simulink model "Filtro_teste_corrente_constante"  (R2014a)
settings: Solver=ode45  StartTime=0.0  StopTime=0.08  MaxStep=1e-6  RelTol=1e-3
libraries: powerlib x36, dsparch4 x4, powerlib_meascontrol x4, simulink x2, sps_avr x1
settings Model: Creator=JPSOLIV  LastModifiedBy=Joao
settings SolverCC: AlgebraicLoopSolver=LineSearch
settings DebuggingCC: MergeDetectMultiDrivingBlocksExec=error

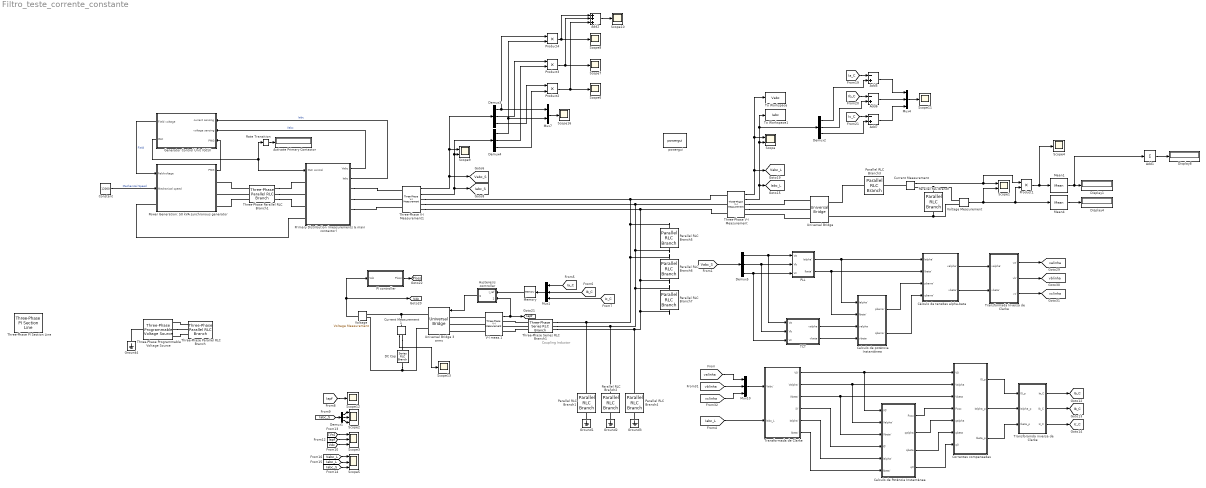
== system Filtro_teste_corrente_constante ==
  note: Coupling Inductor
  Activate Primary Contactor : Display
      settings: SampleTime=1e-2
  Add1 : Sum  Inputs=+
  Add2 : Sum  Inputs=+++
  Add5 : Sum  Inputs=-+
  Add6 : Sum  Inputs=-+
  Add7 : Sum  Inputs=-+
  Calculo de Potência Instantânea : Subsystem
  Calculo de potência Instantânea : Subsystem
  Constant : Constant  Value=12000
  Correntes compensadas : Subsystem
  Current Measurement : powerlib/Measurements/Current Measurement  PhasorSimulation=off  OutputType=Complex  PSBequivalent=0
  Current Measurement1 : powerlib/Measurements/Current Measurement  PhasorSimulation=off  OutputType=Complex  PSBequivalent=0
  Cálculo de tensões alpha-beta : Subsystem
  DC Cap : powerlib/Elements/Series RLC Branch  LConnTagsString=__new0  RConnTagsString=__new0  BranchType=C  Resistance=1  Inductance=1e-3  SetiL0=off  InitialCurrent=0  Capacitance=100e-6  Setx0=off  InitialVoltage=4000  Measurements=None
  Demux{1..5} (5 alike) : Demux  Outputs=3
  Display1 : Display
  Display4 : Display
  Display8 : Display
  Generator Control Unit (GCU) : Subsystem
      mask Display: image(imread('power_aircraft_distribution_GCU.jpg','jpg'))
  Ground{1..4} (4 alike) : powerlib/Elements/Ground  LConnTagsString=a
  Hysteresis controller : Subsystem
  Mean1 : powerlib_meascontrol/Measurements/Mean  Freq=400  Vinit=0  Ts=0
  Mean4 : powerlib_meascontrol/Measurements/Mean  Freq=400  Vinit=0  Ts=0
  Memory : Memory
  Mux1 : Mux  Inputs=3
  Mux10 : Mux  Inputs=3
  Mux4 : Mux  Inputs=3
  Mux7 : Mux  Inputs=2
  PI controller : Subsystem
  PLL : Subsystem
  Parallel RLC Branch : powerlib/Elements/Parallel RLC Branch  LConnTagsString=a  RConnTagsString=__new0  BranchType=RC  Resistance=50  Inductance=1e-3  SetiL0=off  InitialCurrent=0  Capacitance=30e-6  Setx0=off  InitialVoltage=0  Measurements=None
  Parallel RLC Branch1 : powerlib/Elements/Parallel RLC Branch  LConnTagsString=a  RConnTagsString=__new0  BranchType=RC  Resistance=10e3  Inductance=1e-3  SetiL0=off  InitialCurrent=0  Capacitance=3.9789e-08  Setx0=off  InitialVoltage=0  Measurements=None
  Parallel RLC Branch2 : powerlib/Elements/Parallel RLC Branch  LConnTagsString=a  RConnTagsString=__new0  BranchType=RC  Resistance=10e3  Inductance=1e-3  SetiL0=off  InitialCurrent=0  Capacitance=3.9789e-08  Setx0=off  InitialVoltage=0  Measurements=None
  Parallel RLC Branch3 : powerlib/Elements/Parallel RLC Branch  LConnTagsString=a  RConnTagsString=__new0  BranchType=L  Resistance=1  Inductance=10e-3  SetiL0=off  InitialCurrent=0  Capacitance=30e-6  Setx0=off  InitialVoltage=0  Measurements=None
  Parallel RLC Branch4 : powerlib/Elements/Parallel RLC Branch  LConnTagsString=a  RConnTagsString=__new0  BranchType=RC  Resistance=10e3  Inductance=1e-3  SetiL0=off  InitialCurrent=0  Capacitance=3.9789e-08  Setx0=off  InitialVoltage=0  Measurements=None
  Parallel RLC Branch5 : powerlib/Elements/Parallel RLC Branch  LConnTagsString=a  RConnTagsString=__new0  BranchType=C  Resistance=10e3  Inductance=1e-3  SetiL0=off  InitialCurrent=0  Capacitance=.1e-6  Setx0=off  InitialVoltage=0  Measurements=None
  Parallel RLC Branch6 : powerlib/Elements/Parallel RLC Branch  LConnTagsString=a  RConnTagsString=__new0  BranchType=C  Resistance=10e3  Inductance=1e-3  SetiL0=off  InitialCurrent=0  Capacitance=.1e-6  Setx0=off  InitialVoltage=0  Measurements=None
  Parallel RLC Branch7 : powerlib/Elements/Parallel RLC Branch  LConnTagsString=a  RConnTagsString=__new0  BranchType=C  Resistance=10e3  Inductance=1e-3  SetiL0=off  InitialCurrent=0  Capacitance=.1e-6  Setx0=off  InitialVoltage=0  Measurements=None
  Power Generation: 50 kVA synchronous generator : Subsystem
      mask Display: image(imread('power_aircraft_distribution_APU_Generator.jpg','jpg'))
  Primary Distribution (measurements & main contactor) : Subsystem
  Product{1..4} (4 alike) : Product
  Rate Transition : RateTransition  OutPortSampleTimeOpt=Inherit  OutPortSampleTime=Ts
  Scope : Scope  NumInputPorts=2
      settings: YMin=-200~-25  YMax=200~25
  Scope1 : Scope  NumInputPorts=2
      settings: YMin=-0.00561601~0  YMax=20~500
  Scope{4,6..8,10..13,16} (9 alike) : Scope
      Scope10 settings: YMin=-2000  YMax=16000  SaveName=ScopeData18
      Scope11 settings: YMin=-60  YMax=60  SaveName=ScopeData11
      Scope12 settings: YMin=-150  YMax=200  SaveName=ScopeData12
      Scope13 settings: YMin=-20  YMax=70  SaveName=ScopeData31
      Scope16 settings: YMin=-250  YMax=450  SaveName=ScopeData17
      Scope4 settings: YMin=0  YMax=8000  SaveName=ScopeData2
      Scope6 settings: YMin=-1000  YMax=6000  SaveName=ScopeData7
      Scope7 settings: YMin=-1000  YMax=6000  SaveName=ScopeData13
      Scope8 settings: YMin=-10000  YMax=15000  SaveName=ScopeData14
  Scope2 : Scope  NumInputPorts=3
      settings: TimeRange=0.015  YMin=-40~-40~-40  YMax=40~40~40  SaveName=Isource  MaxDataPoints=500000
  Scope3 : Scope  NumInputPorts=3
      settings: TimeRange=0.015  YMin=-1~-20~275  YMax=1~20~575  SaveName=Vs_Iapf_Vdc  MaxDataPoints=500000
  Scope5 : Scope  NumInputPorts=3
      settings: TimeRange=0.015  YMin=-200~-6~-10  YMax=200~6~10  SaveName=Vs_Iapf_Vdc1  MaxDataPoints=500000
  Scope9 : Scope  NumInputPorts=2
      settings: YMin=-175~-7  YMax=175~7  SaveName=ScopeData9
  TCT : Subsystem
  Three-Phase PI Section Line : powerlib/Elements/Three-Phase PI Section Line  LConnTagsString=a|b|c  RConnTagsString=A|B|C  Frequency=400  Resistances=[ 0.01273 0.3864]  Inductances="[ 0.9337e-3  4.1264e-3]"  Capacitances=[12.74e-9 7.751e-9]  Length=0.005
  Three-Phase Parallel RLC Branch : powerlib/Elements/Three-Phase Parallel RLC Branch  LConnTagsString=A|B|C  RConnTagsString=A|B|C  BranchType=RL  Resistance=0.0367e-3  Inductance=6e-6  Capacitance=1e-6  Measurements=None
  Three-Phase Parallel RLC Branch1 : powerlib/Elements/Three-Phase Parallel RLC Branch  LConnTagsString=A|B|C  RConnTagsString=A|B|C  BranchType=RL  Resistance=0.367  Inductance=6e-3  Capacitance=1e-6  Measurements=None
  Three-Phase Programmable Voltage Source : powerlib/Electrical Sources/Three-Phase Programmable Voltage Source  PositiveSequence="[115*sqrt(3)  0 400]"  VariationEntity=None  VariationType=Table of time-amplitude pairs  VariationTypeAlt=Step  VariationStep=0.5  VariationRate=10  VariationMagnitude=0.3  VariationFrequency=2  VariationTiming=[1 2]  VariationPhaseA=off  Amplitudes=[1 0.8 1.2 1.0]  TimeValues=[0 0.1 0.15 0.2]  HarmonicGeneration=off  HarmonicA=[3 0.2 -25 0]  HarmonicB=[2 0.15 35 2]  Timing="[0.05  3]"  BusType=swing  Pref=0  Qref=0  Qmin=-inf  Qmax=inf
  Three-Phase Series RLC Branch1 : powerlib/Elements/Three-Phase Series RLC Branch  LConnTagsString=A|B|C  RConnTagsString=A|B|C  BranchType=L  Resistance=1e9  Inductance=5e-4  Capacitance=.2e-3  Measurements=None
  Three-Phase V-I Measurement : powerlib/Measurements/Three-Phase V-I Measurement  VoltageMeasurement=phase-to-ground  SetLabelV=off  LabelV=Vabc  Vpu=off  VpuLL=off  CurrentMeasurement=yes  SetLabelI=off  LabelI=Iabc  Ipu=off  Pbase=100e6  Vbase=500e3  OutputType=Complex  PhasorSimulation=off  PSBequivalent=0
  Three-Phase V-I Measurement1 : powerlib/Measurements/Three-Phase V-I Measurement  VoltageMeasurement=phase-to-ground  SetLabelV=off  LabelV=Vabc  Vpu=off  VpuLL=off  CurrentMeasurement=yes  SetLabelI=off  LabelI=Iabc  Ipu=off  Pbase=100e6  Vbase=500e3  OutputType=Complex  PhasorSimulation=off  PSBequivalent=0
  To Workspace : ToWorkspace  VariableName=Vabc  SaveFormat=Structure With Time  SampleTime=-1
  To Workspace1 : ToWorkspace  VariableName=Iabc  SaveFormat=Structure With Time  SampleTime=-1
  Transforamda inversa de Clarke : Subsystem
  Transformada Inversa de Clarke : Subsystem
  Transformada de Clarke : Subsystem
  Universal Bridge : powerlib/Power Electronics/Universal Bridge  Arms=3  SnubberResistance=1e5  SnubberCapacitance=inf  Device=Diodes  Ron=1e-3  Lon=0  ForwardVoltages="[  0  0  ]"  ForwardVoltage=0  GTOparameters=[ 10e-6 , 20e-6 ]  IGBTparameters=[ 1e-6 , 2e-6 ]  Measurements=None  Measurements_2=None  converterType=Rectifier
  Universal Bridge 3 arms : powerlib/Power Electronics/Universal Bridge  Arms=3  SnubberResistance=10000  SnubberCapacitance=inf  Device=IGBT / Diodes  Ron=1e-4  Lon=0  ForwardVoltages="[  1  1  ]"  ForwardVoltage=.8  GTOparameters=[ 10e-6 , 20e-6 ]  IGBTparameters=[ 1e-6 , 2e-6 ]  Measurements=None  Measurements_2=None  converterType=Rectifier
  V-I meas.1 : powerlib/Measurements/Three-Phase V-I Measurement  VoltageMeasurement=phase-to-phase  SetLabelV=on  LabelV=Vnm  Vpu=off  VpuLL=off  CurrentMeasurement=yes  SetLabelI=off  LabelI=Iabc  Ipu=off  Pbase=100e6  Vbase=500e3  OutputType=Complex  PhasorSimulation=off  PSBequivalent=0
  Voltage : powerlib/Measurements/Voltage Measurement  PhasorSimulation=off  OutputType=Complex  PSBequivalent=0
  Voltage Measurement : powerlib/Measurements/Voltage Measurement  PhasorSimulation=off  OutputType=Complex  PSBequivalent=0
  powergui : powerlib/powergui  Priority=1  SimulationMode=Discrete  SolverType=Tustin  SampleTime=1e-7  frequency=60  SPID=off  DisableSnubberDevices=off  DisableRonSwitches=off  DisableVfSwitches=off  SwTol=0  Interpol=off  DisplayEquations=off  Ts=100  methode=off  frequencyindice=400  Pbase=100e6  ErrMax=1e-4  Iterations=50  UnitsV=kV  UnitsW=MW  FunctionMessages=off  echomessages=off  HookPort=off  EnableUseOfTLC=off  x0status=blocks  RestoreLinks=warning  ResistiveCurrentMeasurement=off  Frange=[0:2:500]  Ylog=off  Xlog=on  ShowGrid=off  save=off  variable=ZData  structure=0  ZoomFFT=off  StartTime=0.0  cycles=1  DisplayStyle=1  fundamental=60  FreqAxis=off  MaxFrequency=1000  frequencyindicesteady=1  RmsSteady=1  display=off
  tag scope: Ia_C=global, Iabc_L=global, Iabc_S=global, Iapf=global, Ib_C=global, Ic_C=global, Ploss=global, Vabc_L=global, Vabc_S=global, Vdc=global, valinha=global, vblinha=global, vclinha=global
  wires:
  Three-Phase V-I Measurement/1 -> [Vabc_L], To Workspace/1, Scope/1
  Three-Phase V-I Measurement/2 -> [Iabc_L], Demux2/1, To Workspace1/1, Scope/2
  [Ia_C] -> Add5/1
  [Ib_C] -> Add6/1
  [Ic_C] -> Add7/1
  Demux2/1 -> Add5/2
  Demux2/2 -> Add6/2
  Demux2/3 -> Add7/2
  Add6/1 -> Mux4/2
  Mux4/1 -> Scope11/1
  Add7/1 -> Mux4/3
  Add5/1 -> Mux4/1
  Current Measurement/1 -> Product1/1, Scope1/1
  Voltage Measurement/1 -> Scope1/2, Product1/2, Mean4/1
  Product1/1 -> Scope4/1, Mean1/1
  Mean1/1 -> Add1/1, Display1/1
  Mean4/1 -> Display4/1
  Add1/1 -> Display8/1
  Three-Phase V-I Measurement1/1 -> [Vabc_S], Demux3/1, Scope9/1
  Three-Phase V-I Measurement1/2 -> [Iabc_S], Demux4/1, Scope9/2
  Demux3/1 -> Mux7/1, Product4/1
  Mux7/1 -> Scope16/1
  Transformada de Clarke/1(V0') -> Calculo de Potência Instantânea/1(V0'), Correntes compensadas/1(V0)
  Correntes compensadas/2(Ialpha_p) -> Transforamda inversa de Clarke/2(Ialpha_p)
  Correntes compensadas/3(Ibeta_p) -> Transforamda inversa de Clarke/3(Ibeta_p)
  Voltage/1 -> [Vdc], PI controller/1(Vdc)
  PI controller/1(Ploss) -> [Ploss]
  Transforamda inversa de Clarke/1(Ia_C) -> [Ia_C]
  Transforamda inversa de Clarke/2(Ib_C) -> [Ib_C]
  Transforamda inversa de Clarke/3(Ic_C) -> [Ic_C]
  [Iapf] -> Scope12/1
  Demux1/1 -> Scope2/1
  Demux1/2 -> Scope2/2
  Demux1/3 -> Scope2/3
  [Iabc_S] -> Demux1/1
  [Vs] -> Scope3/1
  [Vdc] -> Scope3/3
  [Iapf] -> Scope3/2
  [Vabc_L] -> Scope5/1
  [Iabc_S] -> Scope5/3
  [Iabc_L] -> Scope5/2
  Product2/1 -> Add2/3, Scope6/1
  Power Generation: 50 kVA synchronous generator/1(PMG) -> Generator Control Unit (GCU)/3(PMG)
  Generator Control Unit (GCU)/1(Field voltage) -> Power Generation: 50 kVA synchronous generator/1(fieldvoltage)  "Field"
  Primary Distribution (measurements & main contactor)/1(Vabc) -> Generator Control Unit (GCU)/2(voltage sensing)  "Vabc"
  Primary Distribution (measurements & main contactor)/2(Iabc) -> Generator Control Unit (GCU)/1(current sensing)  "Iabc"
  Generator Control Unit (GCU)/2(GLC) -> Primary Distribution (measurements & main contactor)/1(GLC control), Rate Transition/1
  Constant/1 -> Power Generation: 50 kVA synchronous generator/2(Mechanical speed)  "Mechanical Speed"
  Rate Transition/1 -> Activate Primary Contactor/1
  V-I meas.1/1 -> Hysteresis controller/2(I_meas), [Iapf]
  Mux1/1 -> Memory/1
  Hysteresis controller/1(g) -> Universal Bridge 3 arms/1
  [Ia_C] -> Mux1/1
  [Ib_C] -> Mux1/2
  [Ic_C] -> Mux1/3
  Memory/1 -> Hysteresis controller/1(I_ref)
  Product3/1 -> Add2/2, Scope7/1
  Demux4/1 -> Mux7/2, Product4/2
  Demux3/2 -> Product3/1
  Demux4/2 -> Product3/2
  Demux3/3 -> Product2/1
  Demux4/3 -> Product2/2
  Product4/1 -> Scope8/1, Add2/1
  Add2/1 -> Scope10/1
  [Vabc_S] -> Demux5/1
  [valinha] -> Mux10/1
  [vblinha] -> Mux10/2
  [vclinha] -> Mux10/3
  Mux10/1 -> Transformada de Clarke/1(Vabc')
  [Iabc_L] -> Transformada de Clarke/2(Iabc_L)
  Transformada de Clarke/2(Valpha') -> Calculo de Potência Instantânea/2(Valpha'), Correntes compensadas/2(Valpha)
  Transformada de Clarke/3(Vbeta') -> Calculo de Potência Instantânea/3(Vbeta'), Correntes compensadas/3(Vbeta)
  Transformada de Clarke/4(i0') -> Calculo de Potência Instantânea/4(I0')
  Transformada de Clarke/5(Ialpha') -> Calculo de Potência Instantânea/5(Ialpha')
  Transformada de Clarke/6(Ibeta') -> Calculo de Potência Instantânea/6(Ibeta')
  Calculo de Potência Instantânea/1(Posc) -> Correntes compensadas/4(Posc)
  Calculo de Potência Instantânea/2(qalpha) -> Correntes compensadas/5(qalpha)
  Calculo de Potência Instantânea/3(qbeta) -> Correntes compensadas/6(qbeta)
  Calculo de Potência Instantânea/4(q0) -> Correntes compensadas/7(q0)
  Correntes compensadas/1(I0_p) -> Transforamda inversa de Clarke/1(I0_p)
  Demux5/1 -> PLL/1(Va), TCT/1(Va)
  Demux5/2 -> PLL/2(Vb), TCT/2(Vb)
  Demux5/3 -> PLL/3(Vc), TCT/3(Vc)
  TCT/1(valpha) -> Calculo de potência Instantânea/3(valpha)
  TCT/2(vbeta) -> Calculo de potência Instantânea/4(vbeta)
  Calculo de potência Instantânea/2(qbarra') -> Cálculo de tensões alpha-beta/4(qbarra')
  PLL/1(Ialpha') -> Calculo de potência Instantânea/1(Ialpha'), Cálculo de tensões alpha-beta/1(Ialpha')
  PLL/2(Ibeta') -> Calculo de potência Instantânea/2(Ibeta'), Cálculo de tensões alpha-beta/2(Ibeta')
  Calculo de potência Instantânea/1(pbarra') -> Cálculo de tensões alpha-beta/3(pbarra')
  Cálculo de tensões alpha-beta/1(valpha') -> Transformada Inversa de Clarke/1(valpha')
  Cálculo de tensões alpha-beta/2(vbeta') -> Transformada Inversa de Clarke/2(vbeta')
  Transformada Inversa de Clarke/1(va') -> [valinha]
  Transformada Inversa de Clarke/2(vb') -> [vblinha]
  Transformada Inversa de Clarke/3(vc') -> [vclinha]
  Current Measurement1/1 -> Scope13/1
  connections:
  Parallel RLC Branch/RConn1 -- Universal Bridge/RConn2 -- Voltage Measurement/LConn2
  Three-Phase V-I Measurement/RConn1 -- Universal Bridge/LConn1
  Current Measurement/RConn1 -- Voltage Measurement/LConn1 -- Parallel RLC Branch/LConn1
  Parallel RLC Branch3/RConn1 -- Universal Bridge/RConn1
  Three-Phase V-I Measurement1/RConn2 -- Three-Phase V-I Measurement/LConn2 -- Parallel RLC Branch5/RConn1 -- Three-Phase Series RLC Branch1/RConn2 -- Parallel RLC Branch2/LConn1 -- Parallel RLC Branch7/LConn1
  Current Measurement/LConn1 -- Parallel RLC Branch3/LConn1
  Three-Phase V-I Measurement/RConn2 -- Universal Bridge/LConn2
  Universal Bridge/LConn3 -- Three-Phase V-I Measurement/RConn3
  Three-Phase V-I Measurement1/RConn3 -- Three-Phase V-I Measurement/LConn3 -- Parallel RLC Branch6/RConn1 -- Parallel RLC Branch4/LConn1 -- Three-Phase Series RLC Branch1/RConn3 -- Parallel RLC Branch7/RConn1
  Three-Phase V-I Measurement1/RConn1 -- Parallel RLC Branch1/LConn1 -- Three-Phase Series RLC Branch1/RConn1 -- Parallel RLC Branch6/LConn1 -- Parallel RLC Branch5/LConn1 -- Three-Phase V-I Measurement/LConn1
  Universal Bridge 3 arms/RConn1 -- Current Measurement1/LConn1 -- Voltage/LConn1
  Universal Bridge 3 arms/RConn2 -- Voltage/LConn2 -- DC Cap/RConn1
  V-I meas.1/LConn2 -- Universal Bridge 3 arms/LConn2
  V-I meas.1/LConn1 -- Universal Bridge 3 arms/LConn1
  V-I meas.1/LConn3 -- Universal Bridge 3 arms/LConn3
  Ground1/LConn1 -- Parallel RLC Branch1/RConn1
  Ground2/LConn1 -- Parallel RLC Branch2/RConn1
  Ground3/LConn1 -- Parallel RLC Branch4/RConn1
  Three-Phase Parallel RLC Branch1/RConn3 -- Primary Distribution (measurements & main contactor)/LConn3
  Three-Phase Parallel RLC Branch1/LConn1 -- Power Generation: 50 kVA synchronous generator/RConn1
  Three-Phase Parallel RLC Branch1/LConn2 -- Power Generation: 50 kVA synchronous generator/RConn2
  Power Generation: 50 kVA synchronous generator/LConn1 -- Primary Distribution (measurements & main contactor)/LConn4
  Three-Phase Parallel RLC Branch1/RConn2 -- Primary Distribution (measurements & main contactor)/LConn2
  Three-Phase Parallel RLC Branch1/LConn3 -- Power Generation: 50 kVA synchronous generator/RConn3
  Three-Phase Parallel RLC Branch1/RConn1 -- Primary Distribution (measurements & main contactor)/LConn1
  Three-Phase Series RLC Branch1/LConn2 -- V-I meas.1/RConn2
  Three-Phase Series RLC Branch1/LConn1 -- V-I meas.1/RConn1
  Three-Phase Series RLC Branch1/LConn3 -- V-I meas.1/RConn3
  Primary Distribution (measurements & main contactor)/RConn2 -- Three-Phase V-I Measurement1/LConn2
  Primary Distribution (measurements & main contactor)/RConn1 -- Three-Phase V-I Measurement1/LConn1
  Primary Distribution (measurements & main contactor)/RConn3 -- Three-Phase V-I Measurement1/LConn3
  Three-Phase Programmable Voltage Source/RConn2 -- Three-Phase Parallel RLC Branch/LConn2
  Three-Phase Parallel RLC Branch/LConn1 -- Three-Phase Programmable Voltage Source/RConn1
  Three-Phase Parallel RLC Branch/LConn3 -- Three-Phase Programmable Voltage Source/RConn3
  Three-Phase Programmable Voltage Source/LConn1 -- Ground4/LConn1
  Current Measurement1/RConn1 -- DC Cap/LConn1

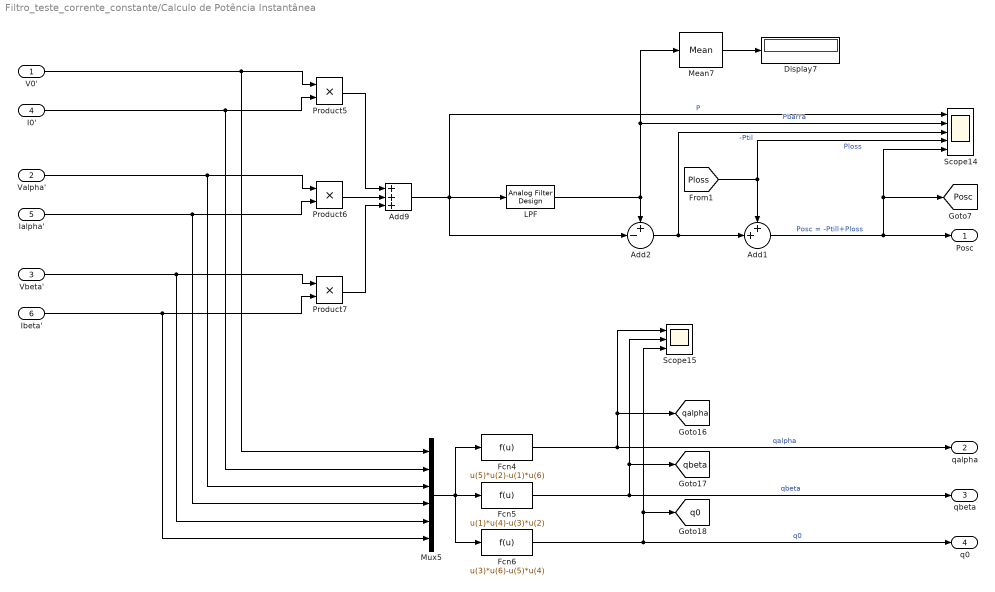
== system Filtro_teste_corrente_constante/Calculo de Potência Instantânea ==
  V0' : Inport
  Valpha' : Inport  Port=2
  Vbeta' : Inport  Port=3
  I0' : Inport  Port=4
  Ialpha' : Inport  Port=5
  Ibeta' : Inport  Port=6
  Add1 : Sum  Inputs=++|
  Add2 : Sum  Inputs=+-|
  Add9 : Sum  Inputs=+++
  Display7 : Display
  Fcn4 : Fcn  Expr=u(5)*u(2)-u(1)*u(6)
  Fcn5 : Fcn  Expr=u(1)*u(4)-u(3)*u(2)
  Fcn6 : Fcn  Expr=u(3)*u(6)-u(5)*u(4)
  LPF : dsparch4/Analog Filter Design  method=Butterworth  filttype=Lowpass  N=5  Wlo=2*pi*100  Whi=80  Rp=2  Rs=40
  Mean7 : powerlib_meascontrol/Measurements/Mean  Freq=400  Vinit=0  Ts=0
  Mux5 : Mux  Inputs=6
  Product5 : Product
  Product6 : Product
  Product7 : Product
  Scope14 : Scope  NumInputPorts=5
      settings: YMin=-250~0~-1750~-30~-1750  YMax=1750~1700~500~90~500  SaveName=ScopeData15
  Scope15 : Scope  NumInputPorts=3
      settings: YMin=0~0~-5000  YMax=105000~5000~105000  SaveName=ScopeData16
  Posc : Outport
  qalpha : Outport  Port=2
  qbeta : Outport  Port=3
  q0 : Outport  Port=4
  tag scope: Posc=global, q0=global, qalpha=global, qbeta=global
  wires:
  [Ploss] -> Scope14/4, Add1/1  "Ploss"
  Add1/1 -> Posc/1, [Posc], Scope14/5  "Posc = -Ptill+Ploss"
  Add2/1 -> Scope14/3, Add1/2  "-Ptil"
  Fcn4/1 -> Scope15/1, [qalpha], qalpha/1  "qalpha"
  Valpha'/1 -> Product6/1, Mux5/3
  LPF/1 -> Mean7/1, Scope14/2, Add2/1  "Pbarra"
  V0'/1 -> Product5/1, Mux5/1
  Ibeta'/1 -> Product7/2, Mux5/6
  Product6/1 -> Add9/2
  Vbeta'/1 -> Product7/1, Mux5/5
  I0'/1 -> Product5/2, Mux5/2
  Ialpha'/1 -> Product6/2, Mux5/4
  Product5/1 -> Add9/1
  Mux5/1 -> Fcn4/1, Fcn6/1, Fcn5/1
  Add9/1 -> Scope14/1, LPF/1, Add2/2  "P"
  Mean7/1 -> Display7/1
  Fcn6/1 -> q0/1, Scope15/3, [q0]  "q0"
  Product7/1 -> Add9/3
  Fcn5/1 -> Scope15/2, [qbeta], qbeta/1  "qbeta"

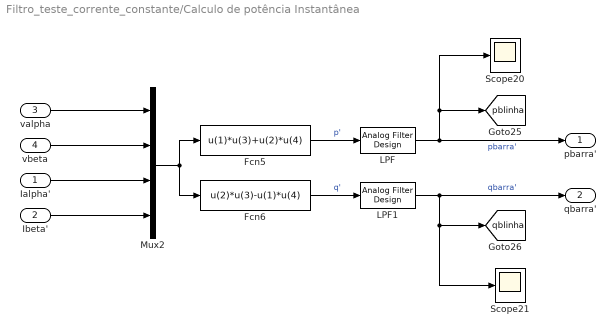
== system Filtro_teste_corrente_constante/Calculo de potência Instantânea ==
  Ialpha' : Inport
  Ibeta' : Inport  Port=2
  valpha : Inport  Port=3
  vbeta : Inport  Port=4
  Fcn5 : Fcn  Expr=u(1)*u(3)+u(2)*u(4)
  Fcn6 : Fcn  Expr=u(2)*u(3)-u(1)*u(4)
  LPF : dsparch4/Analog Filter Design  method=Butterworth  filttype=Lowpass  N=5  Wlo=2*pi*100  Whi=80  Rp=2  Rs=40
  LPF1 : dsparch4/Analog Filter Design  method=Butterworth  filttype=Lowpass  N=5  Wlo=2*pi*100  Whi=80  Rp=2  Rs=40
  Mux2 : Mux
  Scope20 : Scope
      settings: YMin=-50  YMax=250  SaveName=ScopeData25
  Scope21 : Scope
      settings: YMin=0  YMax=80  SaveName=ScopeData26
  pbarra' : Outport
  qbarra' : Outport  Port=2
  tag scope: pblinha=global, qblinha=global
  wires:
  Ibeta'/1 -> Mux2/4
  Ialpha'/1 -> Mux2/3
  LPF1/1 -> Scope21/1, [qblinha], qbarra'/1  "qbarra'"
  LPF/1 -> pbarra'/1, Scope20/1, [pblinha]  "pbarra'"
  Mux2/1 -> Fcn6/1, Fcn5/1
  Fcn6/1 -> LPF1/1  "q'"
  Fcn5/1 -> LPF/1  "p'"
  vbeta/1 -> Mux2/2
  valpha/1 -> Mux2/1

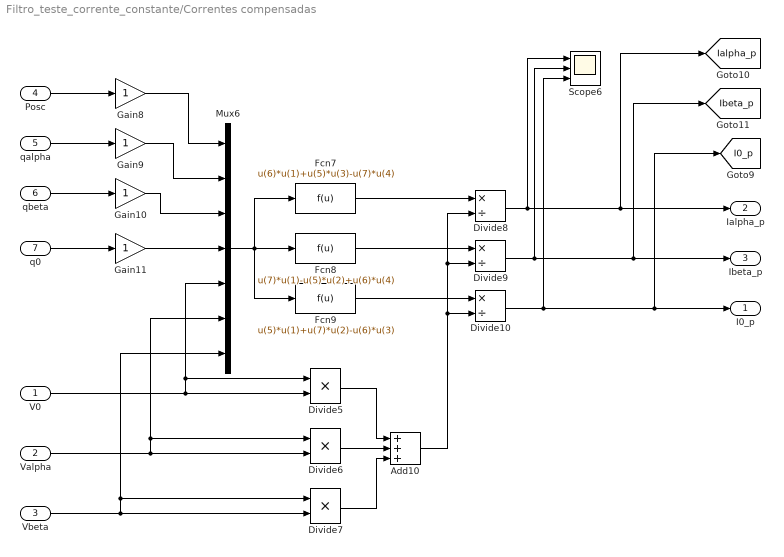
== system Filtro_teste_corrente_constante/Correntes compensadas ==
  V0 : Inport
  Valpha : Inport  Port=2
  Vbeta : Inport  Port=3
  Posc : Inport  Port=4
  qalpha : Inport  Port=5
  qbeta : Inport  Port=6
  q0 : Inport  Port=7
  Add10 : Sum  Inputs=+++
  Divide10 : Product  Inputs=*/
  Divide5 : Product  Inputs=**
  Divide6 : Product  Inputs=**
  Divide7 : Product  Inputs=**
  Divide8 : Product  Inputs=*/
  Divide9 : Product  Inputs=*/
  Fcn7 : Fcn  Expr=u(6)*u(1)+u(5)*u(3)-u(7)*u(4)
  Fcn8 : Fcn  Expr=u(7)*u(1)-u(5)*u(2)+u(6)*u(4)
  Fcn9 : Fcn  Expr=u(5)*u(1)+u(7)*u(2)-u(6)*u(3)
  Gain{8..11} (4 alike) : Gain
  Mux6 : Mux  Inputs=7
  Scope6 : Scope  NumInputPorts=3
      settings: YMin=-25~-20~-5e-10  YMax=20~40~4e-10  SaveName=ScopeData6
  I0_p : Outport
  Ialpha_p : Outport  Port=2
  Ibeta_p : Outport  Port=3
  tag scope: I0_p=global, Ialpha_p=global, Ibeta_p=global
  wires:
  Valpha/1 -> Mux6/6, Divide6/1, Divide6/2
  Divide9/1 -> Scope6/2, [Ibeta_p], Ibeta_p/1
  Fcn9/1 -> Divide10/1
  Mux6/1 -> Fcn7/1, Fcn9/1, Fcn8/1
  Posc/1 -> Gain8/1
  Vbeta/1 -> Mux6/7, Divide7/1, Divide7/2
  Gain11/1 -> Mux6/4
  qalpha/1 -> Gain9/1
  q0/1 -> Gain11/1
  qbeta/1 -> Gain10/1
  Divide8/1 -> Scope6/1, [Ialpha_p], Ialpha_p/1
  Fcn7/1 -> Divide8/1
  Gain10/1 -> Mux6/3
  Gain9/1 -> Mux6/2
  Fcn8/1 -> Divide9/1
  Divide7/1 -> Add10/3
  Gain8/1 -> Mux6/1
  Divide6/1 -> Add10/2
  Divide5/1 -> Add10/1
  V0/1 -> Mux6/5, Divide5/1, Divide5/2
  Add10/1 -> Divide10/2, Divide9/2, Divide8/2
  Divide10/1 -> Scope6/3, [I0_p], I0_p/1

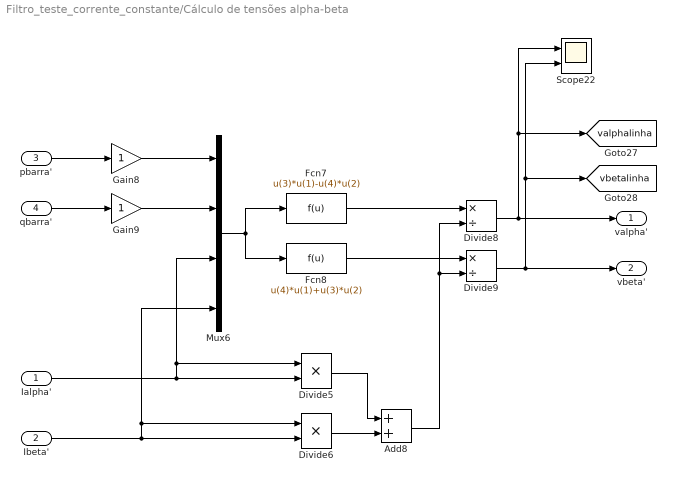
== system Filtro_teste_corrente_constante/Cálculo de tensões alpha-beta ==
  Ialpha' : Inport
  Ibeta' : Inport  Port=2
  pbarra' : Inport  Port=3
  qbarra' : Inport  Port=4
  Add8 : Sum
  Divide5 : Product  Inputs=**
  Divide6 : Product  Inputs=**
  Divide8 : Product  Inputs=*/
  Divide9 : Product  Inputs=*/
  Fcn7 : Fcn  Expr=u(3)*u(1)-u(4)*u(2)
  Fcn8 : Fcn  Expr=u(4)*u(1)+u(3)*u(2)
  Gain8 : Gain
  Gain9 : Gain
  Mux6 : Mux
  Scope22 : Scope  NumInputPorts=2
      settings: YMin=-250~-250  YMax=250~250  SaveName=ScopeData27
  valpha' : Outport
  vbeta' : Outport  Port=2
  tag scope: valphalinha=global, vbetalinha=global
  wires:
  pbarra'/1 -> Gain8/1
  Divide5/1 -> Add8/1
  Divide6/1 -> Add8/2
  Gain8/1 -> Mux6/1
  Fcn8/1 -> Divide9/1
  Mux6/1 -> Fcn8/1, Fcn7/1
  qbarra'/1 -> Gain9/1
  Divide8/1 -> valpha'/1, Scope22/1, [valphalinha]
  Fcn7/1 -> Divide8/1
  Gain9/1 -> Mux6/2
  Divide9/1 -> Scope22/2, [vbetalinha], vbeta'/1
  Ibeta'/1 -> Mux6/4, Divide6/1, Divide6/2
  Ialpha'/1 -> Mux6/3, Divide5/1, Divide5/2
  Add8/1 -> Divide9/2, Divide8/2

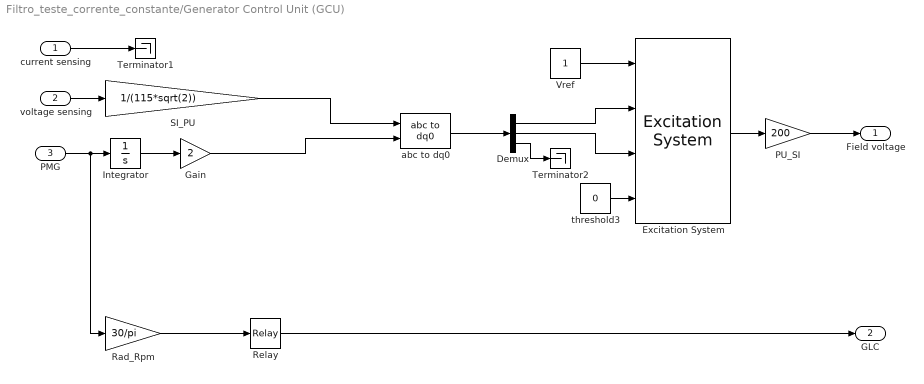
== system Filtro_teste_corrente_constante/Generator Control Unit (GCU) ==
  current sensing : Inport
  voltage sensing : Inport  Port=2
  PMG : Inport  Port=3
  Demux : Demux  Outputs=3
  Excitation System : sps_avr/Excitation System  tr=20e-3  reg=[ 300, 0.001 ]  exc=[ 1, 0 ]  tgr=[ 0, 0 ]  damp=[ 0.001, 0.1 ]  sat=[ 0, 0 ]  lim=[ -2, 2, 0 ]  v0=[1 0]
  Gain : Gain  Gain=2
  Integrator : Integrator
  PU_SI : Gain  Gain=200
  Rad_Rpm : Gain  Gain=30/pi
  Relay : Relay  OnSwitchValue=9000  OffSwitchValue=8900
  SI_PU : Gain  Gain=1/(115*sqrt(2))
  Terminator1 : Terminator
  Terminator2 : Terminator
  Vref : Constant
  abc to dq0 : powerlib_meascontrol/Transformations/abc to dq0  Alignment=90 degrees behind phase A axis
  threshold3 : Constant  Value=0
  Field voltage : Outport
  GLC : Outport  Port=2
  wires:
  Relay/1 -> GLC/1
  Demux/3 -> Terminator2/1
  current sensing/1 -> Terminator1/1
  threshold3/1 -> Excitation System/4
  Vref/1 -> Excitation System/1
  Rad_Rpm/1 -> Relay/1
  PU_SI/1 -> Field voltage/1
  Excitation System/1 -> PU_SI/1
  SI_PU/1 -> abc to dq0/1
  Demux/2 -> Excitation System/3
  Demux/1 -> Excitation System/2
  abc to dq0/1 -> Demux/1
  Integrator/1 -> Gain/1
  voltage sensing/1 -> SI_PU/1
  PMG/1 -> Rad_Rpm/1, Integrator/1
  Gain/1 -> abc to dq0/2

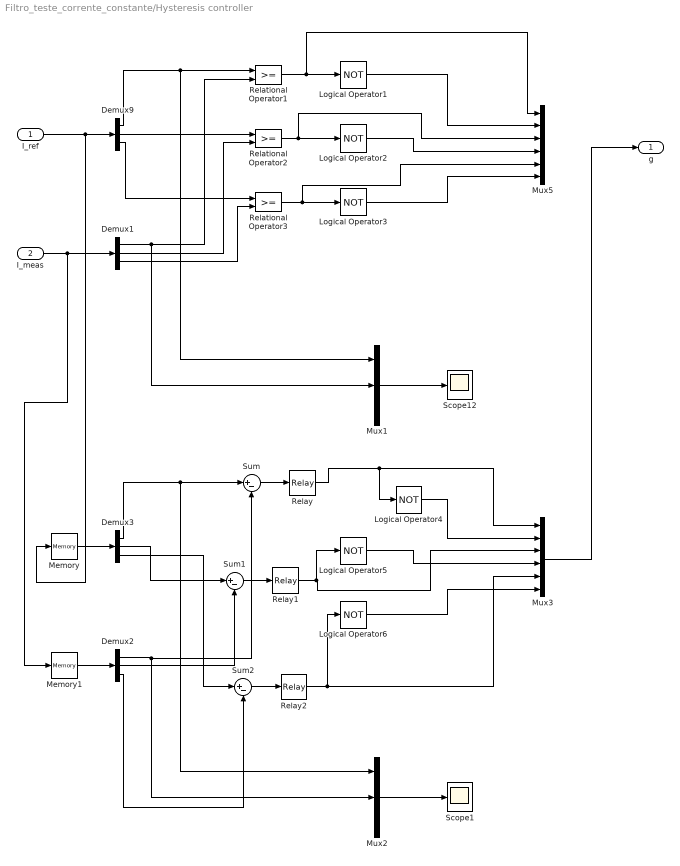
== system Filtro_teste_corrente_constante/Hysteresis controller ==
  I_ref : Inport
  I_meas : Inport  Port=2
  Demux{1..3,9} (4 alike) : Demux  Outputs=3
  Logical Operator{1..6} (6 alike) : Logic  Operator=NOT  AllPortsSameDT=off  OutDataTypeStr=boolean
  Memory : Memory
  Memory1 : Memory
  Mux1 : Mux  Inputs=3
  Mux2 : Mux  Inputs=3
  Mux3 : Mux  Inputs=6
  Mux5 : Mux  Inputs=6
  Relational Operator1 : RelationalOperator  OutDataTypeStr=boolean
  Relational Operator2 : RelationalOperator  OutDataTypeStr=boolean
  Relational Operator3 : RelationalOperator  OutDataTypeStr=boolean
  Relay : Relay  OnSwitchValue=0.05  OffSwitchValue=-0.05  OutDataTypeStr=Inherit: Inherit via back propagation
  Relay1 : Relay  OnSwitchValue=0.05  OffSwitchValue=-0.05  OutDataTypeStr=Inherit: Inherit via back propagation
  Relay2 : Relay  OnSwitchValue=0.05  OffSwitchValue=-0.05  OutDataTypeStr=Inherit: Inherit via back propagation
  Scope1 : Scope
      settings: YMin=-9  YMax=7  SaveName=ScopeData30
  Scope12 : Scope
      settings: YMin=-1.2e+45  YMax=1e+44  SaveName=ScopeData8
  Sum : Sum  Inputs=|+-
  Sum1 : Sum  Inputs=|+-
  Sum2 : Sum  Inputs=|+-
  g : Outport
  wires:
  Relational Operator1/1 -> Logical Operator1/1, Mux5/1
  Relational Operator2/1 -> Logical Operator2/1, Mux5/3
  Relational Operator3/1 -> Logical Operator3/1, Mux5/5
  Demux9/1 -> Mux1/1, Relational Operator1/1
  Logical Operator1/1 -> Mux5/2
  Logical Operator2/1 -> Mux5/4
  Logical Operator3/1 -> Mux5/6
  Demux9/2 -> Relational Operator2/1
  Demux1/1 -> Mux1/2, Relational Operator1/2
  Demux1/2 -> Relational Operator2/2
  Demux1/3 -> Relational Operator3/2
  I_ref/1 -> Memory/1, Demux9/1
  I_meas/1 -> Memory1/1, Demux1/1
  Demux9/3 -> Relational Operator3/1
  Mux1/1 -> Scope12/1
  Relay1/1 -> Logical Operator5/1, Mux3/3
  Demux3/1 -> Mux2/1, Sum/1
  Logical Operator4/1 -> Mux3/2
  Logical Operator5/1 -> Mux3/4
  Logical Operator6/1 -> Mux3/6
  Mux3/1 -> g/1
  Demux2/1 -> Sum/2, Mux2/2
  Memory/1 -> Demux3/1
  Memory1/1 -> Demux2/1
  Mux2/1 -> Scope1/1
  Sum/1 -> Relay/1
  Relay/1 -> Logical Operator4/1, Mux3/1
  Demux3/2 -> Sum1/1
  Demux2/2 -> Sum1/2
  Sum1/1 -> Relay1/1
  Demux3/3 -> Sum2/1
  Sum2/1 -> Relay2/1
  Demux2/3 -> Sum2/2
  Relay2/1 -> Logical Operator6/1, Mux3/5

== system Filtro_teste_corrente_constante/PI controller ==
  Vdc : Inport
  Constant : Constant  Value=400
  Discrete PID Controller : simulink/Continuous/PID Controller  Controller=PI  TimeDomain=Discrete-time  SampleTime=1e-6  IntegratorMethod=Forward Euler  FilterMethod=Forward Euler  Form=Parallel  P=1  I=0.1  D=0  N=100  InitialConditionSource=internal  InitialConditionForIntegrator=0  InitialConditionForFilter=0  ExternalReset=none  LimitOutput=off  UpperSaturationLimit=inf  LowerSaturationLimit=-inf  LinearizeAsGain=off  AntiWindupMode=none  Kb=1  TrackingMode=off  Kt=1  PParamMin=[]  PParamMax=[]  IParamMin=[]  IParamMax=[]  DParamMin=[]  DParamMax=[]  NParamMin=[]  NParamMax=[]  KbParamMin=[]  KbParamMax=[]  KtParamMin=[]  KtParamMax=[]  POutMin=[]  POutMax=[]  IOutMin=[]  IOutMax=[]  DOutMin=[]  DOutMax=[]  NOutMin=[]  NOutMax=[]  KbOutMin=[]  KbOutMax=[]  KtOutMin=[]  KtOutMax=[]  IntegratorOutMin=[]  IntegratorOutMax=[]  FilterOutMin=[]  FilterOutMax=[]  SumOutMin=[]  SumOutMax=[]  SumI1OutMin=[]  SumI1OutMax=[]  SumI2OutMin=[]  SumI2OutMax=[]  SumI3OutMin=[]  SumI3OutMax=[]  SumDOutMin=[]  SumDOutMax=[]  SaturationOutMin=[]  SaturationOutMax=[]  IntegratorContinuousStateAttributes=''  IntegratorStateMustResolveToSignalObject=off  IntegratorRTWStateStorageClass=Auto  FilterContinuousStateAttributes=''  FilterStateMustResolveToSignalObject=off  FilterRTWStateStorageClass=Auto
  LPF : dsparch4/Analog Filter Design  method=Butterworth  filttype=Lowpass  N=5  Wlo=2*pi*50  Whi=80  Rp=2  Rs=40
  Scope1 : Scope  NumInputPorts=2
      settings: TimeRange=0.025  YMin=-50~-50  YMax=450~450  SaveName=psb3phPWM1_str1  MaxDataPoints=500000
  Sum : Sum  Inputs=|-+
  Ploss : Outport
  wires:
  Vdc/1 -> Sum/1, Scope1/1
  Sum/1 -> LPF/1, Scope1/2
  LPF/1 -> Discrete PID Controller/1
  Constant/1 -> Sum/2
  Discrete PID Controller/1 -> Ploss/1

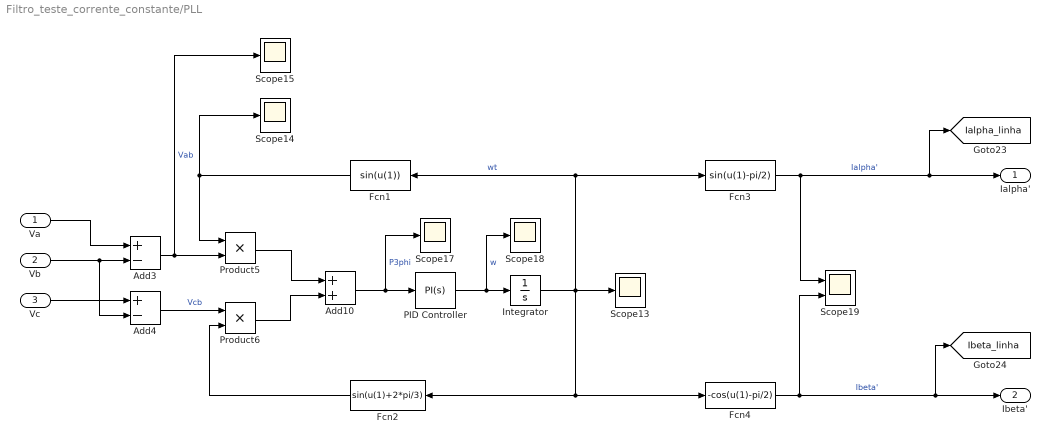
== system Filtro_teste_corrente_constante/PLL ==
  Va : Inport
  Vb : Inport  Port=2
  Vc : Inport  Port=3
  Add10 : Sum
  Add3 : Sum  Inputs=+-
  Add4 : Sum  Inputs=+-
  Fcn1 : Fcn  Expr=sin(u(1))
  Fcn2 : Fcn  Expr=sin(u(1)+2*pi/3)
  Fcn3 : Fcn  Expr=sin(u(1)-pi/2)
  Fcn4 : Fcn  Expr=-cos(u(1)-pi/2)
  Integrator : Integrator
  PID Controller : simulink/Continuous/PID Controller  Controller=PI  TimeDomain=Continuous-time  SampleTime=-1  IntegratorMethod=Forward Euler  FilterMethod=Forward Euler  Form=Parallel  P=30  I=1  D=0  N=100  InitialConditionSource=internal  InitialConditionForIntegrator=0  InitialConditionForFilter=0  ExternalReset=none  LimitOutput=off  UpperSaturationLimit=inf  LowerSaturationLimit=-inf  LinearizeAsGain=on  AntiWindupMode=none  Kb=1  TrackingMode=off  Kt=1  PParamMin=[]  PParamMax=[]  IParamMin=[]  IParamMax=[]  DParamMin=[]  DParamMax=[]  NParamMin=[]  NParamMax=[]  KbParamMin=[]  KbParamMax=[]  KtParamMin=[]  KtParamMax=[]  POutMin=[]  POutMax=[]  IOutMin=[]  IOutMax=[]  DOutMin=[]  DOutMax=[]  NOutMin=[]  NOutMax=[]  KbOutMin=[]  KbOutMax=[]  KtOutMin=[]  KtOutMax=[]  IntegratorOutMin=[]  IntegratorOutMax=[]  FilterOutMin=[]  FilterOutMax=[]  SumOutMin=[]  SumOutMax=[]  SumI1OutMin=[]  SumI1OutMax=[]  SumI2OutMin=[]  SumI2OutMax=[]  SumI3OutMin=[]  SumI3OutMax=[]  SumDOutMin=[]  SumDOutMax=[]  SaturationOutMin=[]  SaturationOutMax=[]  IntegratorContinuousStateAttributes=''  IntegratorStateMustResolveToSignalObject=off  IntegratorRTWStateStorageClass=Auto  FilterContinuousStateAttributes=''  FilterStateMustResolveToSignalObject=off  FilterRTWStateStorageClass=Auto
  Product5 : Product
  Product6 : Product
  Scope{13..15,17..18} (5 alike) : Scope
      Scope13 settings: YMin=0  YMax=120  SaveName=ScopeData19
      Scope14 settings: YMin=-0.2  YMax=0.2  SaveName=ScopeData20
      Scope15 settings: YMin=-500  YMax=500  SaveName=ScopeData21
      Scope17 settings: YMin=-300  YMax=300  SaveName=ScopeData22
      Scope18 settings: YMin=0  YMax=7000  SaveName=ScopeData23
  Scope19 : Scope  NumInputPorts=2
      settings: YMin=-1~-1  YMax=1~1  SaveName=ScopeData24
  Ialpha' : Outport
  Ibeta' : Outport  Port=2
  tag scope: Ialpha_linha=global, Ibeta_linha=global
  wires:
  Va/1 -> Add3/1
  Add3/1 -> Scope15/1, Product5/2  "Vab"
  Vc/1 -> Add4/1
  Fcn3/1 -> Ialpha'/1, [Ialpha_linha], Scope19/1  "Ialpha'"
  Fcn1/1 -> Scope14/1, Product5/1
  Fcn2/1 -> Product6/2
  Integrator/1 -> Fcn2/1, Fcn4/1, Fcn1/1, Fcn3/1, Scope13/1  "wt"
  Product6/1 -> Add10/2
  Vb/1 -> Add4/2, Add3/2
  Product5/1 -> Add10/1
  Add4/1 -> Product6/1  "Vcb"
  PID Controller/1 -> Scope18/1, Integrator/1  "w"
  Add10/1 -> Scope17/1, PID Controller/1  "P3phi"
  Fcn4/1 -> Scope19/2, Ibeta'/1, [Ibeta_linha]  "Ibeta'"

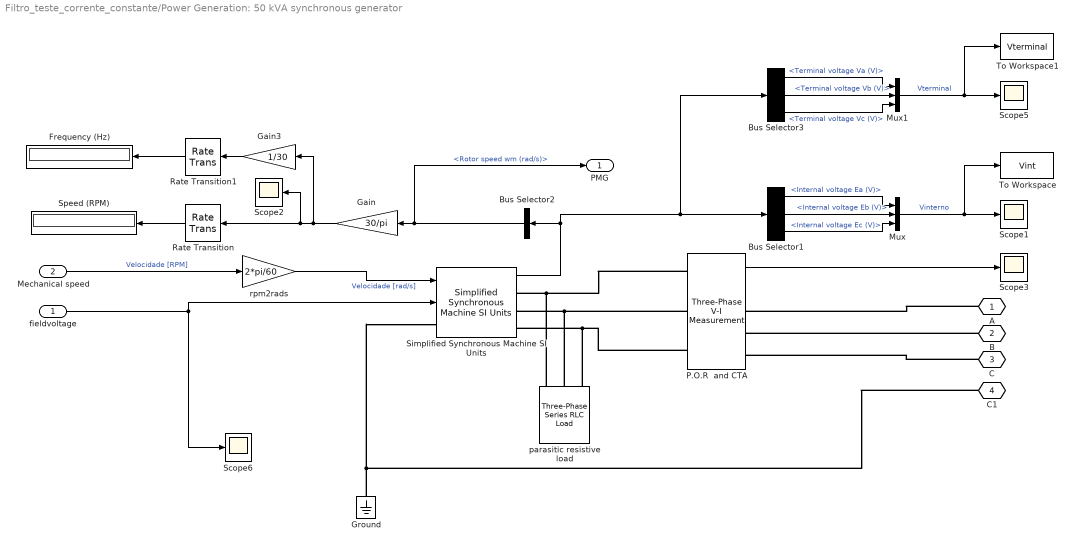
== system Filtro_teste_corrente_constante/Power Generation: 50 kVA synchronous generator ==
  fieldvoltage : Inport
  Mechanical speed : Inport  Port=2
  Bus Selector1 : BusSelector  OutputSignals=Internal voltage Ea (V),Internal voltage Eb (V),Internal voltage Ec (V)
  Bus Selector2 : BusSelector  OutputSignals=Rotor speed wm (rad/s)
  Bus Selector3 : BusSelector  OutputSignals=Terminal voltage Va (V),Terminal voltage Vb (V),Terminal voltage Vc (V)
  Frequency (Hz) : Display
      settings: SampleTime=1e-2
  Gain : Gain  Gain=30/pi
  Gain3 : Gain  Gain=1/30
  Ground : powerlib/Elements/Ground  LConnTagsString=a
  Mux : Mux  Inputs=3
  Mux1 : Mux  Inputs=3
  P.O.R  and CTA : powerlib/Measurements/Three-Phase V-I Measurement  VoltageMeasurement=phase-to-ground  SetLabelV=off  LabelV=Vabc  Vpu=off  VpuLL=off  CurrentMeasurement=yes  SetLabelI=off  LabelI=Iabc  Ipu=off  Pbase=100e6  Vbase=500e3  OutputType=Complex  PhasorSimulation=off  PSBequivalent=0
  Rate Transition : RateTransition  OutPortSampleTimeOpt=Inherit  OutPortSampleTime=Ts
  Rate Transition1 : RateTransition  OutPortSampleTimeOpt=Inherit  OutPortSampleTime=Ts
  Scope{1..3,5..6} (5 alike) : Scope
      Scope1 settings: TimeRange=0.01  YMin=-110  YMax=120  Decimation=100  SampleTime=1e-3
      Scope2 settings: TimeRange=1  YMin=11400  YMax=12600  SaveName=ScopeData3  Decimation=100  SampleTime=1e-3
      Scope3 settings: TimeRange=0.005  YMin=-200  YMax=200  Decimation=100  SampleTime=1e-3
      Scope5 settings: TimeRange=0.005  YMin=-225  YMax=200  SaveName=ScopeData4  Decimation=100  SampleTime=1e-3
      Scope6 settings: TimeRange=0.005  YMin=380  YMax=420  SaveName=ScopeData5  Decimation=100  SampleTime=1e-3
  Simplified Synchronous Machine SI Units : powerlib/Machines/Simplified Synchronous Machine SI Units  ConnectionType=4-wire Y  MechanicalLoad=Speed w  MeasurementBus=off  NominalParameters=[50e3 200 400]  Mechanical=[0.02 0 2]  InternalRL="[0.0204  0.08104e-3]"  InitialConditions=[0,0 0,0,0 0,0,0]  Units=1  LoadFlowParameters=[1,0,0,0,0]  TsPowergui=0  TsBlock=-1  BusType=PV  Pref=0  Qref=0  Qmin=-inf  Qmax=+inf  PLF=0  QLF=0
  Speed (RPM) : Display
      settings: SampleTime=1e-2
  To Workspace : ToWorkspace  VariableName=Vint  SaveFormat=Structure With Time  SampleTime=-1
  To Workspace1 : ToWorkspace  VariableName=Vterminal  SaveFormat=Structure With Time  SampleTime=-1
  parasitic resistive load : powerlib/Elements/Three-Phase Series RLC Load  LConnTagsString=A|B|C  Configuration=Y (grounded)  NominalVoltage=200  NominalFrequency=400  ActivePower=5000  InductivePower=0  CapacitivePower=0  Measurements=None  LoadType=constant Z
  rpm2rads : Gain  Gain=2*pi/60
  A : PMIOPort  Tag=PMCPort  Port=1  Side=Right
  B : PMIOPort  Tag=PMCPort  Port=2  Side=Right
  C : PMIOPort  Tag=PMCPort  Port=3  Side=Right
  C1 : PMIOPort  Tag=PMCPort  Port=4  Side=Left
  PMG : Outport
  wires:
  Simplified Synchronous Machine SI Units/1 -> Bus Selector3/1, Bus Selector1/1, Bus Selector2/1
  fieldvoltage/1 -> Scope6/1, Simplified Synchronous Machine SI Units/2
  Bus Selector2/1 -> PMG/1, Gain/1  "<Rotor speed wm (rad/s)>"
  Gain/1 -> Gain3/1, Scope2/1, Rate Transition/1
  Gain3/1 -> Rate Transition1/1
  Mechanical speed/1 -> rpm2rads/1  "Velocidade [RPM]"
  Rate Transition/1 -> Speed (RPM)/1
  Rate Transition1/1 -> Frequency (Hz)/1
  Bus Selector1/2 -> Mux/2  "<Internal voltage Eb (V)>"
  Bus Selector1/3 -> Mux/3  "<Internal voltage Ec (V)>"
  Bus Selector1/1 -> Mux/1  "<Internal voltage Ea (V)>"
  Mux/1 -> Scope1/1, To Workspace/1  "Vinterno"
  P.O.R  and CTA/1 -> Scope3/1
  Bus Selector3/2 -> Mux1/2  "<Terminal voltage Vb (V)>"
  Bus Selector3/3 -> Mux1/3  "<Terminal voltage Vc (V)>"
  Bus Selector3/1 -> Mux1/1  "<Terminal voltage Va (V)>"
  Mux1/1 -> To Workspace1/1, Scope5/1  "Vterminal"
  rpm2rads/1 -> Simplified Synchronous Machine SI Units/1  "Velocidade [rad/s]"
  connections:
  Ground/LConn1 -- C1/RConn1 -- Simplified Synchronous Machine SI Units/LConn1
  P.O.R  and CTA/LConn1 -- parasitic resistive load/LConn1 -- Simplified Synchronous Machine SI Units/RConn1
  P.O.R  and CTA/LConn2 -- parasitic resistive load/LConn2 -- Simplified Synchronous Machine SI Units/RConn2
  P.O.R  and CTA/LConn3 -- parasitic resistive load/LConn3 -- Simplified Synchronous Machine SI Units/RConn3
  A/RConn1 -- P.O.R  and CTA/RConn1
  B/RConn1 -- P.O.R  and CTA/RConn2
  C/RConn1 -- P.O.R  and CTA/RConn3

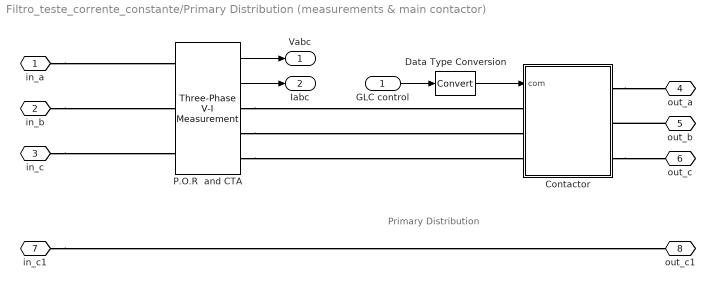
== system Filtro_teste_corrente_constante/Primary Distribution (measurements & main contactor) ==
  note: Primary Distribution
  GLC control : Inport
  Contactor : Subsystem
  Data Type Conversion : DataTypeConversion
  P.O.R  and CTA : powerlib/Measurements/Three-Phase V-I Measurement  VoltageMeasurement=phase-to-ground  SetLabelV=off  LabelV=Vabc  Vpu=off  VpuLL=off  CurrentMeasurement=yes  SetLabelI=off  LabelI=Iabc  Ipu=off  Pbase=100e6  Vbase=500e3  OutputType=Complex  PhasorSimulation=off  PSBequivalent=0
  in_a : PMIOPort  Port=1  Side=Left
  in_b : PMIOPort  Port=2  Side=Left
  in_c : PMIOPort  Port=3  Side=Left
  out_a : PMIOPort  Port=4  Side=Right
  out_b : PMIOPort  Port=5  Side=Right
  out_c : PMIOPort  Port=6  Side=Right
  in_c1 : PMIOPort  Port=7  Side=Left
  out_c1 : PMIOPort  Port=8  Side=Right
  Vabc : Outport
  Iabc : Outport  Port=2
  wires:
  GLC control/1 -> Data Type Conversion/1
  P.O.R  and CTA/1 -> Vabc/1
  P.O.R  and CTA/2 -> Iabc/1
  Data Type Conversion/1 -> Contactor/1(com)
  connections:
  in_a/RConn1 -- P.O.R  and CTA/LConn1
  in_b/RConn1 -- P.O.R  and CTA/LConn2
  in_c/RConn1 -- P.O.R  and CTA/LConn3
  P.O.R  and CTA/RConn1 -- Contactor/LConn1
  P.O.R  and CTA/RConn2 -- Contactor/LConn2
  P.O.R  and CTA/RConn3 -- Contactor/LConn3
  Contactor/RConn1 -- out_a/RConn1
  out_b/RConn1 -- Contactor/RConn2
  Contactor/RConn3 -- out_c/RConn1
  in_c1/RConn1 -- out_c1/RConn1

== system Filtro_teste_corrente_constante/TCT ==
  Va : Inport
  Vb : Inport  Port=2
  Vc : Inport  Port=3
  Demux7 : Demux  Outputs=3
  Gain1 : Gain  Gain=sqrt(2/3)
  Gain3 : Gain  Gain=[1/sqrt(2), 1/sqrt(2), 1/sqrt(2); 1, -1/2, -1/2; 0, sqrt(3)/2, -sqrt(3)/2]  Multiplication=Matrix(K*u)
  Mux2 : Mux  Inputs=3
  valpha : Outport
  vbeta : Outport  Port=2
  wires:
  Gain3/1 -> Demux7/1  "Valphabeta0"
  Gain1/1 -> Gain3/1
  Mux2/1 -> Gain1/1
  Va/1 -> Mux2/1
  Vb/1 -> Mux2/2
  Vc/1 -> Mux2/3
  Demux7/2 -> valpha/1
  Demux7/3 -> vbeta/1

== system Filtro_teste_corrente_constante/Transforamda inversa de Clarke ==
  I0_p : Inport
  Ialpha_p : Inport  Port=2
  Ibeta_p : Inport  Port=3
  Fcn1 : Fcn  Expr=sqrt(2/3)*(1/sqrt(2)*u(1)+u(2))
  Fcn2 : Fcn  Expr=sqrt(2/3)*(1/sqrt(2)*u(1)-1/2*u(2)+sqrt(3)/2*u(3))
  Fcn3 : Fcn  Expr=sqrt(2/3)*(1/sqrt(2)*u(1)-1/2*u(2)-sqrt(3)/2*u(3))
  Mux1 : Mux  Inputs=3
  Mux2 : Mux  Inputs=3
  Mux3 : Mux  Inputs=3
  Scope10 : Scope  NumInputPorts=4
      settings: YMin=-2.25~-3~-2.5~-6e-10  YMax=3~0~3.5~1.5e-10  SaveName=ScopeData10
  Ia_C : Outport
  Ib_C : Outport  Port=2
  Ic_C : Outport  Port=3
  wires:
  Fcn2/1 -> Ib_C/1, Scope10/2  "Ib_C"
  Mux2/1 -> Fcn2/1
  Mux1/1 -> Fcn1/1
  Fcn3/1 -> Ic_C/1, Scope10/3  "Ic_C"
  Ibeta_p/1 -> Mux3/3, Mux1/3, Mux2/3
  Fcn1/1 -> Ia_C/1, Scope10/1  "Ia_C"
  Mux3/1 -> Fcn3/1
  Ialpha_p/1 -> Mux3/2, Mux2/2, Mux1/2
  I0_p/1 -> Scope10/4, Mux2/1, Mux3/1, Mux1/1

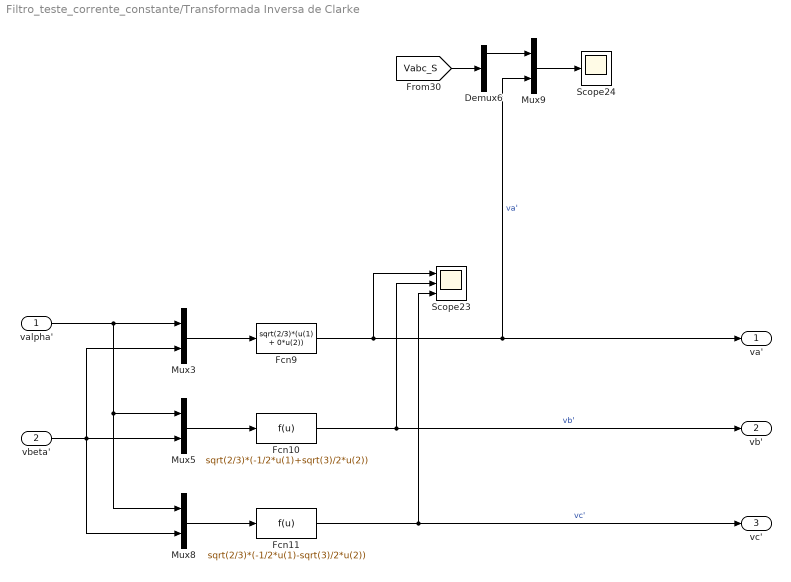
== system Filtro_teste_corrente_constante/Transformada Inversa de Clarke ==
  valpha' : Inport
  vbeta' : Inport  Port=2
  Demux6 : Demux  Outputs=3
  Fcn10 : Fcn  Expr=sqrt(2/3)*(-1/2*u(1)+sqrt(3)/2*u(2))
  Fcn11 : Fcn  Expr=sqrt(2/3)*(-1/2*u(1)-sqrt(3)/2*u(2))
  Fcn9 : Fcn  Expr=sqrt(2/3)*(u(1) + 0*u(2))
  Mux{3,5,8..9} (4 alike) : Mux  Inputs=2
  Scope23 : Scope  NumInputPorts=3
      settings: YMin=-200~-200~-200  YMax=200~200~200  SaveName=ScopeData28
  Scope24 : Scope
      settings: YMin=-200  YMax=200  SaveName=ScopeData29
  va' : Outport
  vb' : Outport  Port=2
  vc' : Outport  Port=3
  wires:
  Fcn10/1 -> vb'/1, Scope23/2  "vb'"
  Mux9/1 -> Scope24/1
  Demux6/1 -> Mux9/1
  valpha'/1 -> Mux5/1, Mux8/1, Mux3/1
  vbeta'/1 -> Mux3/2, Mux5/2, Mux8/2
  Mux5/1 -> Fcn10/1
  Mux3/1 -> Fcn9/1
  Fcn11/1 -> vc'/1, Scope23/3  "vc'"
  Fcn9/1 -> va'/1, Mux9/2, Scope23/1  "va'"
  Mux8/1 -> Fcn11/1
  [Vabc_S] -> Demux6/1

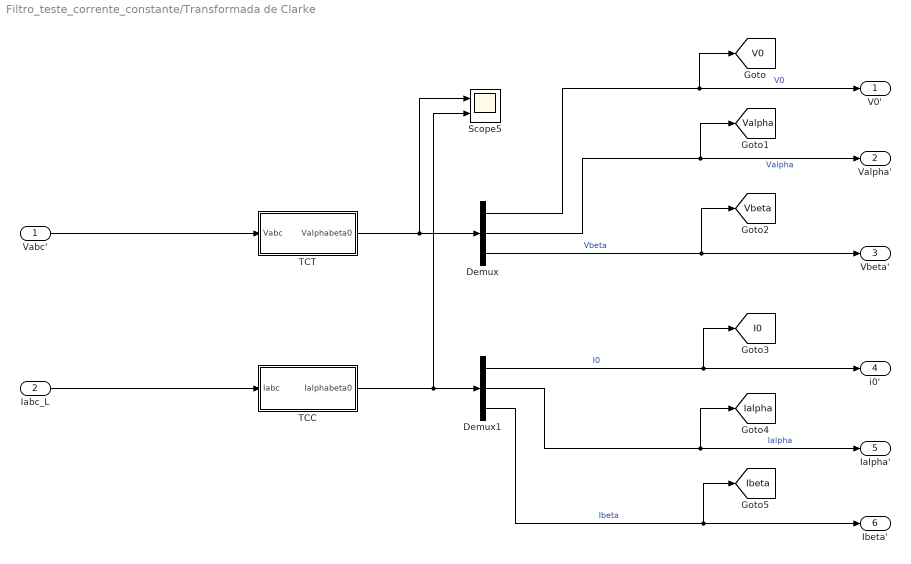
== system Filtro_teste_corrente_constante/Transformada de Clarke ==
  Vabc' : Inport
  Iabc_L : Inport  Port=2
  Demux : Demux  Outputs=3
  Demux1 : Demux  Outputs=3
  Scope5 : Scope  NumInputPorts=2
      settings: YMin=-600~-200  YMax=400~200  SaveName=ScopeData5
  TCC : Subsystem
  TCT : Subsystem
  V0' : Outport
  Valpha' : Outport  Port=2
  Vbeta' : Outport  Port=3
  i0' : Outport  Port=4
  Ialpha' : Outport  Port=5
  Ibeta' : Outport  Port=6
  tag scope: I0=global, Ialpha=global, Ibeta=global, V0=global, Valpha=global, Vbeta=global
  wires:
  TCT/1(Valphabeta0) -> Scope5/1, Demux/1
  Iabc_L/1 -> TCC/1(Iabc)
  Vabc'/1 -> TCT/1(Vabc)
  Demux/3 -> [Vbeta], Vbeta'/1  "Vbeta"
  Demux/2 -> Valpha'/1, [Valpha]  "Valpha"
  Demux/1 -> [V0], V0'/1  "V0"
  Demux1/1 -> [I0], i0'/1  "I0"
  Demux1/2 -> [Ialpha], Ialpha'/1  "Ialpha"
  Demux1/3 -> [Ibeta], Ibeta'/1  "Ibeta"
  TCC/1(Ialphabeta0) -> Scope5/2, Demux1/1

== system Filtro_teste_corrente_constante/Primary Distribution (measurements & main contactor)/Contactor ==
  com : Inport
  Ideal Switch : powerlib/Power Electronics/Ideal Switch  Ron=0.001  Lon=0  IC=0  Rs=1e3  Cs=inf  Measurements=off
  Ideal Switch1 : powerlib/Power Electronics/Ideal Switch  Ron=0.001  Lon=0  IC=0  Rs=1e3  Cs=inf  Measurements=off
  Ideal Switch2 : powerlib/Power Electronics/Ideal Switch  Ron=0.001  Lon=0  IC=0  Rs=1e3  Cs=inf  Measurements=off
  A : PMIOPort  Port=1  Side=Left
  a : PMIOPort  Port=2  Side=Right
  B : PMIOPort  Port=3  Side=Left
  b : PMIOPort  Port=4  Side=Right
  C : PMIOPort  Port=5  Side=Left
  c : PMIOPort  Port=6  Side=Right
  wires:
  com/1 -> Ideal Switch1/1, Ideal Switch2/1, Ideal Switch/1
  connections:
  c/RConn1 -- Ideal Switch2/RConn1
  C/RConn1 -- Ideal Switch2/LConn1
  b/RConn1 -- Ideal Switch1/RConn1
  B/RConn1 -- Ideal Switch1/LConn1
  a/RConn1 -- Ideal Switch/RConn1
  A/RConn1 -- Ideal Switch/LConn1

== system Filtro_teste_corrente_constante/Transformada de Clarke/TCC ==
  Iabc : Inport
  Gain2 : Gain  Gain=sqrt(2/3)
  Gain4 : Gain  Gain=[1/sqrt(2), 1/sqrt(2), 1/sqrt(2); 1, -1/2, -1/2; 0, sqrt(3)/2, -sqrt(3)/2]  Multiplication=Matrix(K*u)
  Ialphabeta0 : Outport
  wires:
  Iabc/1 -> Gain2/1
  Gain4/1 -> Ialphabeta0/1  "Ialphabeta0"
  Gain2/1 -> Gain4/1

== system Filtro_teste_corrente_constante/Transformada de Clarke/TCT ==
  Vabc : Inport
  Gain1 : Gain  Gain=sqrt(2/3)
  Gain3 : Gain  Gain=[1/sqrt(2), 1/sqrt(2), 1/sqrt(2); 1, -1/2, -1/2; 0, sqrt(3)/2, -sqrt(3)/2]  Multiplication=Matrix(K*u)
  Valphabeta0 : Outport
  wires:
  Gain3/1 -> Valphabeta0/1  "Valphabeta0"
  Gain1/1 -> Gain3/1
  Vabc/1 -> Gain1/1
